simulink model "rearvehicle"  (R2020b)
settings: Solver=VariableStepAuto  StartTime=0.01  StopTime=100  RelTol=1e-3
undefined symbols (not defined in the file): aubr, tablebr, vubr
libraries: pid_lib x2, Solver_SF x2
settings Model: Creator=wwcong  LastModifiedBy=85304
settings DataIOCC: ReturnWorkspaceOutputs=off
settings DebuggingCC: ArithmeticOperatorsInVariantConditions=warning
settings SFSimCC: SimUseLocalCustomCode=off  CustomCodeUndefinedFunction=UseInterfaceOnly
settings RTWCC: RTWUseLocalCustomCode=off

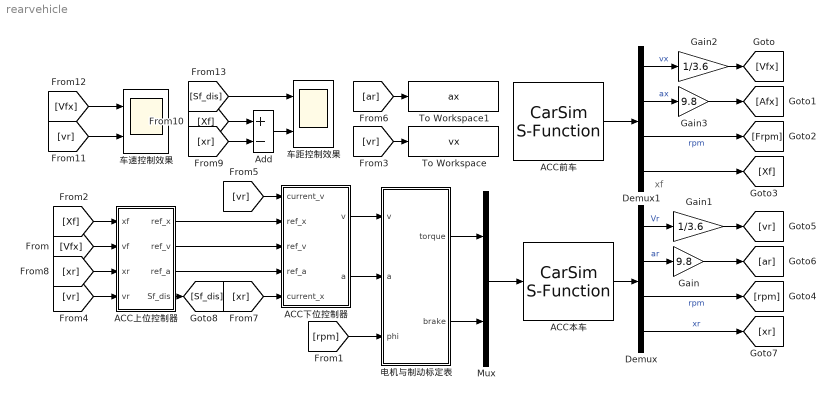
== system rearvehicle ==
  note: xf
  ACC上位控制器 : MATLAB Function  TreatAsAtomicUnit=on
  ACC下位控制器 : Subsystem
  ACC前车 : Solver_SF/CarSim S-Function  Priority=1  SIMFILE=frontvehicel.sim
  ACC本车 : Solver_SF/CarSim S-Function  Priority=1  SIMFILE=rearvehicle.sim
  Add : Sum  Inputs=+-
  Demux : Demux
  Demux1 : Demux
  Gain : Gain  Gain=9.8
  Gain1 : Gain  Gain=1/3.6
  Gain2 : Gain  Gain=1/3.6
  Gain3 : Gain  Gain=9.8
  Mux : Mux  Inputs=2
  To Workspace : ToWorkspace  VariableName=vx  SaveFormat=Timeseries  SampleTime=0.1
  To Workspace1 : ToWorkspace  VariableName=ax  SaveFormat=Timeseries  SampleTime=0.1
  电机与制动标定表 : Subsystem
  车距控制效果 : Scope  NumInputPorts=2
  车速控制效果 : Scope  NumInputPorts=2
  wires:
  ACC本车/1 -> Demux/1
  Mux/1 -> ACC本车/1
  Demux/1 -> Gain1/1  "Vr"
  Demux/2 -> Gain/1  "ar"
  Gain1/1 -> [vr]
  电机与制动标定表/1(torque) -> Mux/1
  电机与制动标定表/2(brake) -> Mux/2
  ACC下位控制器/1(v) -> 电机与制动标定表/1(v)
  ACC下位控制器/2(a) -> 电机与制动标定表/2(a)
  ACC前车/1 -> Demux1/1
  Demux1/4 -> [Xf]
  Demux1/3 -> [Frpm]  "rpm"
  Demux1/1 -> Gain2/1  "vx"
  Gain2/1 -> [Vfx]
  Demux1/2 -> Gain3/1  "ax"
  Gain3/1 -> [Afx]
  [Xf] -> ACC上位控制器/1(xf)
  [Vfx] -> ACC上位控制器/2(vf)
  ACC上位控制器/2(ref_v) -> ACC下位控制器/3(ref_v)
  ACC上位控制器/3(ref_a) -> ACC下位控制器/4(ref_a)
  ACC上位控制器/1(ref_x) -> ACC下位控制器/2(ref_x)
  Demux/3 -> [rpm]  "rpm"
  [rpm] -> 电机与制动标定表/3(phi)
  [vr] -> To Workspace/1
  [vr] -> ACC上位控制器/4(vr)
  [vr] -> ACC下位控制器/1(current_v)
  Gain/1 -> [ar]
  [ar] -> To Workspace1/1
  Demux/4 -> [xr]  "xr"
  [xr] -> ACC下位控制器/5(current_x)
  [xr] -> ACC上位控制器/3(xr)
  [xr] -> Add/2
  [Xf] -> Add/1
  Add/1 -> 车距控制效果/2
  [vr] -> 车速控制效果/2
  [Vfx] -> 车速控制效果/1
  ACC上位控制器/4(Sf_dis) -> [Sf_dis]
  [Sf_dis] -> 车距控制效果/1

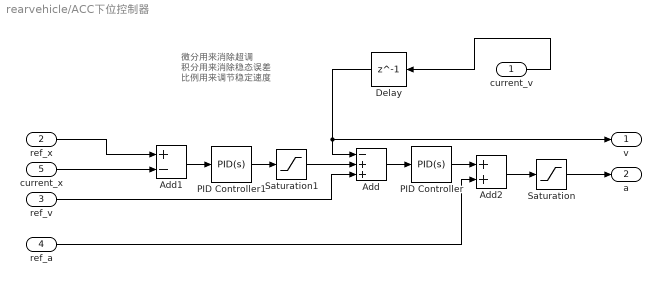
== system rearvehicle/ACC下位控制器 ==
  note: 微分用来消除超调
      | 积分用来消除稳态误差
      | 比例用来调节稳定速度
  current_v : Inport
  ref_x : Inport  Port=2
  ref_v : Inport  Port=3
  ref_a : Inport  Port=4
  current_x : Inport  Port=5
  Add : Sum  Inputs=-++
  Add1 : Sum  Inputs=+-
  Add2 : Sum
  Delay : Delay  DelayLength=1
  PID Controller : pid_lib/PID Controller  Controller=PID  Form=Parallel  TimeDomain=Continuous-time  UseExternalTs=off  SampleTime=-1  IntegratorMethod=Forward Euler  FilterMethod=Forward Euler  ControllerParametersSource=internal  P=1  I=0  D=0.1  UseFilter=on  N=30  TunerSelectOption=Transfer Function Based (PID Tuner App)  InitialConditionSource=internal  InitialConditionForIntegrator=0  InitialConditionForFilter=0  DifferentiatorICPrevScaledInput=0  ExternalReset=none  TrackingMode=off  Kt=1  LimitOutput=off  SatLimitsSource=internal  UpperSaturationLimit=inf  LowerSaturationLimit=-inf  LinearizeAsGain=on  AntiWindupMode=none  Kb=1  POutMin=[]  POutMax=[]  IOutMin=[]  IOutMax=[]  DOutMin=[]  DOutMax=[]  NOutMin=[]  NOutMax=[]  SumOutMin=[]  SumOutMax=[]  SaturationOutMin=[]  SaturationOutMax=[]  PParamMin=[]  PParamMax=[]  IParamMin=[]  IParamMax=[]  DParamMin=[]  DParamMax=[]  NParamMin=[]  NParamMax=[]  KbParamMin=[]  KbParamMax=[]  KtParamMin=[]  KtParamMax=[]  KbOutMin=[]  KbOutMax=[]  KtOutMin=[]  KtOutMax=[]  IntegratorOutMin=[]  IntegratorOutMax=[]  FilterOutMin=[]  FilterOutMax=[]  SumI1OutMin=[]  SumI1OutMax=[]  SumI2OutMin=[]  SumI2OutMax=[]  SumI3OutMin=[]  SumI3OutMax=[]  SumI4OutMin=[]  SumI4OutMax=[]  SumDOutMin=[]  SumDOutMax=[]  DifferentiatorOutMin=[]  DifferentiatorOutMax=[]  FilterDiffOutCoefMin=[]  FilterDiffOutCoefMax=[]  ReciprocalOutMin=[]  ReciprocalOutMax=[]  SumDenOutMin=[]  SumDenOutMax=[]  SumNumOutMin=[]  SumNumOutMax=[]  DivideOutMin=[]  DivideOutMax=[]  UdiffTsProdOutMin=[]  UdiffTsProdOutMax=[]  NTsProdOutMin=[]  NTsProdOutMax=[]  UintegralTsProdOutMin=[]  UintegralTsProdOutMax=[]  UngainTsProdOutMin=[]  UngainTsProdOutMax=[]  IntegratorContinuousStateAttributes=''  IntegratorStateMustResolveToSignalObject=off  IntegratorRTWStateStorageClass=Auto  FilterContinuousStateAttributes=''  FilterStateMustResolveToSignalObject=off  FilterRTWStateStorageClass=Auto  ParallelPVariant=InternalParameters  IdealPVariant=Disabled  IVariant=InternalParameters  DVariant=InternalParameters  IntegratorVariant=Continuous  SatVariant=Disabled  AWVariant=Passthrough  PCopyVariant=Disabled  TRVariant=Disabled  FdbkBlocksVariant=Forward  IdealPFdbkVariant=Disabled  SatFdbkVariant=Disabled  DerivativeFilterVariant=ContFilter  NVariant=InternalParameters  NCopyVariant=Disabled  FilterICVariant=InternalICsFilter  IntegratorICVariant=InternalICs  ExternalResetVariant=Disabled  TRSumVariant=Passthrough  SumFdbkVariant=Disabled  SumVariant=Sum_PID  TsampFilterVariant=InternalTs  TsampNgainVariant=Passthrough  TsampIntegralVariant=Passthrough  ExternalSaturationOutDataTypeStr=Inherit: Same as second input
  PID Controller1 : pid_lib/PID Controller  Controller=PID  Form=Parallel  TimeDomain=Continuous-time  UseExternalTs=off  SampleTime=-1  IntegratorMethod=Forward Euler  FilterMethod=Forward Euler  ControllerParametersSource=internal  P=1  I=0  D=0.1  UseFilter=on  N=30  TunerSelectOption=Transfer Function Based (PID Tuner App)  InitialConditionSource=internal  InitialConditionForIntegrator=0  InitialConditionForFilter=0  DifferentiatorICPrevScaledInput=0  ExternalReset=none  TrackingMode=off  Kt=1  LimitOutput=off  SatLimitsSource=internal  UpperSaturationLimit=inf  LowerSaturationLimit=-inf  LinearizeAsGain=on  AntiWindupMode=none  Kb=1  POutMin=[]  POutMax=[]  IOutMin=[]  IOutMax=[]  DOutMin=[]  DOutMax=[]  NOutMin=[]  NOutMax=[]  SumOutMin=[]  SumOutMax=[]  SaturationOutMin=[]  SaturationOutMax=[]  PParamMin=[]  PParamMax=[]  IParamMin=[]  IParamMax=[]  DParamMin=[]  DParamMax=[]  NParamMin=[]  NParamMax=[]  KbParamMin=[]  KbParamMax=[]  KtParamMin=[]  KtParamMax=[]  KbOutMin=[]  KbOutMax=[]  KtOutMin=[]  KtOutMax=[]  IntegratorOutMin=[]  IntegratorOutMax=[]  FilterOutMin=[]  FilterOutMax=[]  SumI1OutMin=[]  SumI1OutMax=[]  SumI2OutMin=[]  SumI2OutMax=[]  SumI3OutMin=[]  SumI3OutMax=[]  SumI4OutMin=[]  SumI4OutMax=[]  SumDOutMin=[]  SumDOutMax=[]  DifferentiatorOutMin=[]  DifferentiatorOutMax=[]  FilterDiffOutCoefMin=[]  FilterDiffOutCoefMax=[]  ReciprocalOutMin=[]  ReciprocalOutMax=[]  SumDenOutMin=[]  SumDenOutMax=[]  SumNumOutMin=[]  SumNumOutMax=[]  DivideOutMin=[]  DivideOutMax=[]  UdiffTsProdOutMin=[]  UdiffTsProdOutMax=[]  NTsProdOutMin=[]  NTsProdOutMax=[]  UintegralTsProdOutMin=[]  UintegralTsProdOutMax=[]  UngainTsProdOutMin=[]  UngainTsProdOutMax=[]  IntegratorContinuousStateAttributes=''  IntegratorStateMustResolveToSignalObject=off  IntegratorRTWStateStorageClass=Auto  FilterContinuousStateAttributes=''  FilterStateMustResolveToSignalObject=off  FilterRTWStateStorageClass=Auto  ParallelPVariant=InternalParameters  IdealPVariant=Disabled  IVariant=InternalParameters  DVariant=InternalParameters  IntegratorVariant=Continuous  SatVariant=Disabled  AWVariant=Passthrough  PCopyVariant=Disabled  TRVariant=Disabled  FdbkBlocksVariant=Forward  IdealPFdbkVariant=Disabled  SatFdbkVariant=Disabled  DerivativeFilterVariant=ContFilter  NVariant=InternalParameters  NCopyVariant=Disabled  FilterICVariant=InternalICsFilter  IntegratorICVariant=InternalICs  ExternalResetVariant=Disabled  TRSumVariant=Passthrough  SumFdbkVariant=Disabled  SumVariant=Sum_PID  TsampFilterVariant=InternalTs  TsampNgainVariant=Passthrough  TsampIntegralVariant=Passthrough  ExternalSaturationOutDataTypeStr=Inherit: Same as second input
  Saturation : Saturate  UpperLimit=5  LowerLimit=-8
  Saturation1 : Saturate  UpperLimit=10  LowerLimit=-10
  v : Outport
  a : Outport  Port=2
  wires:
  Delay/1 -> v/1, Add/1
  current_x/1 -> Add1/2
  Add/1 -> PID Controller/1
  Add2/1 -> Saturation/1
  PID Controller1/1 -> Saturation1/1
  PID Controller/1 -> Add2/1
  Saturation1/1 -> Add/2
  Saturation/1 -> a/1
  Add1/1 -> PID Controller1/1
  current_v/1 -> Delay/1
  ref_a/1 -> Add2/2
  ref_v/1 -> Add/3
  ref_x/1 -> Add1/1

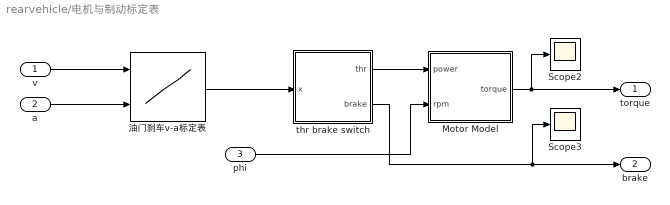
== system rearvehicle/电机与制动标定表 ==
  v : Inport
  a : Inport  Port=2
  phi : Inport  Port=3
  Motor Model : MATLAB Function  TreatAsAtomicUnit=on
  Scope2 : Scope
  Scope3 : Scope
  thr brake switch : MATLAB Function  TreatAsAtomicUnit=on
  油门刹车v-a标定表 : Lookup_n-D  BreakpointsForDimension1=vubr  BreakpointsForDimension2=aubr  Table=tablebr  InternalRulePriority=Speed  RndMeth=Simplest  InputSameDT=on
      settings: InputPortMap=u0,u1
  torque : Outport
  brake : Outport  Port=2
  wires:
  v/1 -> 油门刹车v-a标定表/1
  thr brake switch/2(brake) -> brake/1, Scope3/1
  phi/1 -> Motor Model/2(rpm)
  thr brake switch/1(thr) -> Motor Model/1(power)
  a/1 -> 油门刹车v-a标定表/2
  Motor Model/1(torque) -> torque/1, Scope2/1
  油门刹车v-a标定表/1 -> thr brake switch/1(x)

== matlab function rearvehicle/电机与制动标定表/thr brake switch ==
  data: x input; thr output; brake output
function [thr,brake] = trans(x)

    if(x>0)
        if(x<=1)
        thr=x;
        else
        thr=1;
        end
        brake=0;
    else 
        thr=0;
        brake=-x;
    end
end

== matlab function rearvehicle/电机与制动标定表/Motor Model ==
  data: power input; torque output; rpm input
function torque = fcn(power,rpm)
Tmax=400*power;
    if(rpm<=4523)
        torque=Tmax;
    else 
        torque=Tmax*4523/rpm;
    end
end

== matlab function rearvehicle/ACC上位控制器 ==
  data: ref_x output; xf input; ref_v output; vf input; xr input; ref_a output; vr input; Sf_dis output
function [ref_x,ref_v,ref_a,Sf_dis] = fcn(xf,vf,xr,vr)
dt=1.4;            % 驾驶员跟车时间距
d0=2;              % 驾驶员初始跟车距离
Sf_dis=dt*(vf)+d0; % 安全跟车距离
Cur_dis=xf-xr;     
ref_x=(Cur_dis-Sf_dis)+xr;
ref_v=vf;
t=4;
ref_a=(Cur_dis-Sf_dis)*4/t^2;

% if (abs(vf-vr)>=0.5 && abs(Cur_dis-Sf_dis)>=2 )
%     t=abs(Cur_dis-Sf_dis)/(vf-vr);
% ref_a=(Cur_dis-Sf_dis)*4/t^2;
% elseif(abs(vf-vr)<0.5 && abs(Cur_dis-Sf_dis)>=2 )
%     t=4;
% ref_a=(Cur_dis-Sf_dis)*4/t^2;
% elseif(abs(vf-vr)>=0.5 && abs(Cur_dis-Sf_dis)<2 )
%     t=abs(Cur_dis-Sf_dis)/(vf-vr);
% ref_a=(vf-vr)/t;
% else
% ref_a=(vf-vr);
% end
